simulink model "swingup_polplacement"  (R2020b)
settings: Solver=ode1  StartTime=0.0  StopTime=40  FixedStep=0.01  RelTol=1e-3  EnableMultiTasking=on
values from neighbouring files (symbols this model uses):
  A = A-B*K    [DCMotorODE_up.m]    (also in upright_polplacement.m = [0 0 1 0)
  B = -km * Bold / Rm*gain    [DCMotorODE_up.m]    (also in upright_polplacement.m)
  C = eye(2,4)    [DCMotorODE_up.m]    (also in upright_polplacement.m)
  D = [0;0]    [DCMotorODE_up.m]    (also in upright_polplacement.m = zeros(2,1))
  g = 9.81    [DCMotorODE_up.m]    (also in upright_polplacement.m)
  h = 0.01    [DCMotorODE_up.m]    (also in upright_polplacement.m)
  Jp = mp*Lp^2/3    (= 0.000133128)    [DCMotorODE_up.m]    (also in upright_polplacement.m)
  ke = 0.1    [upright_polplacement.m]
  kt = 0.042    [DCMotorODE_up.m]    (also in upright_polplacement.m)
  l = Lp/2    (= 0.0645)    [DCMotorODE_up.m]    (also in upright_polplacement.m)
  mp = 0.024    [DCMotorODE_up.m]    (also in upright_polplacement.m)
  mr = 0.095    [DCMotorODE_up.m]    (also in upright_polplacement.m)
  r = 0.085    [DCMotorODE_up.m]    (also in upright_polplacement.m)
  Rm = 8.4    [DCMotorODE_up.m]    (also in upright_polplacement.m)
  u_max = 10    [upright_polplacement.m]
undefined symbols (not defined in the file or in its folder): Continuous, Humusoft, K, MF634, Time
libraries: simulink_extras x4, simulink x4, sldrtlib x2, ctrlSharedLib x1, eeLuenbergerObserver x1
settings Model: Creator=rbabuska  LastModifiedBy=zhehanli
settings DataIOCC: LimitDataPoints=on  SaveFormat=Array  SignalLoggingSaveFormat=ModelDataLogs  ReturnWorkspaceOutputs=off
settings OptimizationCC: ExpressionDepthLimit=2147483647  LifeSpan=inf
settings DebuggingCC: UnderspecifiedInitializationDetection=Classic  MergeDetectMultiDrivingBlocksExec=none  FcnCallInpInsideContextMsg=warning  StateNameClashWarn=warning  SFUnexpectedBacktrackingDiag=warning  SFNoUnconditionalDefaultTransitionDiag=warning  SFExecutionAtInitializationDiag=none  ArithmeticOperatorsInVariantConditions=warning
settings HardwareCC: ProdBitPerPointer=32  ProdBitPerSizeT=32  ProdBitPerPtrDiffT=32  ProdLargestAtomicFloat=None  ProdIntDivRoundTo=Undefined  ProdEndianess=Unspecified  ProdWordSize=32  ProdHWDeviceType=32-bit Generic
settings ModelReferenceCC: PropagateSignalLabelsOutOfModel=off
settings SFSimCC: SimUseLocalCustomCode=off  CustomCodeUndefinedFunction=UseInterfaceOnly
settings RTWCC: RTWUseLocalCustomCode=off
settings CodeAppCC: StateflowObjectComments=on
settings GRTTargetCC: TargetLangStandard=C89/C90 (ANSI)  CombineOutputUpdateFcns=off  GRTInterface=on
settings ConfigComp: CovMetricSettings=dw  CovSaveCumulativeToWorkspaceVar=on  CovSaveSingleToWorkspaceVar=on  CovExternalEMLEnable=off  CovSFcnEnable=off

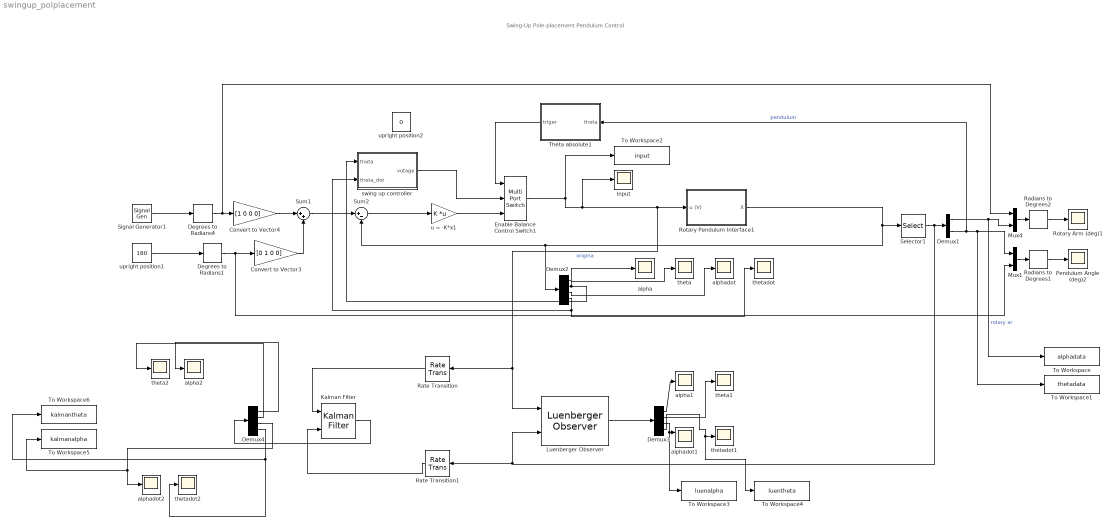
== system swingup_polplacement ==
  note: Swing-Up Pole-placement Pendulum Control
  Convert to Vector3 : Gain  Gain=[0 1 0 0]
  Convert to Vector4 : Gain  Gain=[1 0 0 0]
  Degrees to Radians1 : simulink_extras/Transformations/Degrees to Radians
  Degrees to Radians4 : simulink_extras/Transformations/Degrees to Radians
  Demux1 : Demux  Outputs=2
  Demux2 : Demux
  Demux3 : Demux
  Demux4 : Demux
  Enable Balance Control Switch1 : MultiPortSwitch  DataPortOrder=Zero-based contiguous  Inputs=2  zeroidx=on
  "Input " : Scope
  Kalman Filter : ctrlSharedLib/Kalman Filter  TimeDomain=Continuous-Time  UseCurrentEstimator=on  ModelSource=Individual A, B, C, D matrices  ModelSourceVariable=sys  A=A  B=B  C=C  D=D  NumberOfStates=2  NumberOfInputs=2  NumberOfOutputs=2  InitialEstimateSource=Dialog  X0=[0 0 0 0]  P0=10  UseK=off  UseGH=off  NumberOfProcessNoiseInputs=2  G=1  TimeInvariantG=on  H=0  TimeInvariantH=on  Q=diag([0 0 0.00001 0.00001])  TimeInvariantQ=on  R=0.001  TimeInvariantR=on  N=0  TimeInvariantN=on  AddInputPort=on  AddEnablePort=off  OutputEstimatedY=off  OutputP=off  Ts=h
  Luenberger Observer : eeLuenbergerObserver/Luenberger Observer  StateSpaceType=Continuous-time  Ad=1  Bd=1  Cd=1  Dd=1  A=A  B=B  C=C  D=D  ObserverDesign=Desired eigenvalues  Ld=1  DesiredEigenvalues=[-0.6, -1.5,-10, -20]  x0=[0 0 0 0]  Tsd=0.1  Ts=h
      settings: SourceProductBaseCode=PS
  Mux1 : Mux  Inputs=2
  Mux4 : Mux  Inputs=2
  Pendulum Angle (deg)2 : Scope
  Radians to Degrees1 : simulink_extras/Transformations/Radians to Degrees
  Radians to Degrees2 : simulink_extras/Transformations/Radians to Degrees
  Rate Transition : RateTransition
  Rate Transition1 : RateTransition
  Rotary Arm (deg)1 : Scope
  Rotary Pendulum Interface1 : Subsystem
  Selector1 : Selector  InputPortWidth=4  IndexOptions=Index vector (dialog)  Indices=[1 2]  OutputSizes=1
  Signal Generator1 : SignalGenerator  WaveForm=square  Amplitude=20  Frequency=0.5  Units=rad/sec
  Sum1 : Sum  Inputs=|++
  Sum2 : Sum  Inputs=|+-
  Theta absolute1 : Subsystem
  To Workspace : ToWorkspace  VariableName=alphadata  SaveFormat=Timeseries  SampleTime=h
      settings: Decimation=2
  To Workspace1 : ToWorkspace  VariableName=thetadata  SaveFormat=Timeseries  SampleTime=h
      settings: Decimation=2
  To Workspace2 : ToWorkspace  VariableName=input  SaveFormat=Timeseries  SampleTime=h
      settings: Decimation=2
  To Workspace3 : ToWorkspace  VariableName=luenalpha  SaveFormat=Timeseries  SampleTime=h
      settings: Decimation=2
  To Workspace4 : ToWorkspace  VariableName=luentheta  SaveFormat=Timeseries  SampleTime=h
      settings: Decimation=2
  To Workspace5 : ToWorkspace  VariableName=kalmanalpha  SaveFormat=Timeseries  SampleTime=h
      settings: Decimation=2
  To Workspace6 : ToWorkspace  VariableName=kalmantheta  SaveFormat=Timeseries  SampleTime=h
      settings: Decimation=2
  alpha : Scope
  alpha1 : Scope
  alpha2 : Scope
  alphadot : Scope
  alphadot1 : Scope  NumInputPorts=2
  alphadot2 : Scope
  swing up controller : Subsystem
  theta : Scope
  theta1 : Scope
  theta2 : Scope
  thetadot : Scope
  thetadot1 : Scope
  thetadot2 : Scope
  u = -K*x1 : Gain  Gain=K  Multiplication=Matrix(K*u)
  upright position1 : Constant  Value=180  SampleTime=0
  upright position2 : Constant  Value=0  SampleTime=0
  wires:
  Convert to Vector4/1 -> Sum1/1
  upright position1/1 -> Degrees to Radians1/1
  Demux2/3 -> alphadot/1
  Convert to Vector3/1 -> Sum1/2
  Sum1/1 -> Sum2/1
  u = -K*x1/1 -> Enable Balance Control Switch1/3
  Demux2/1 -> alpha/1
  Degrees to Radians4/1 -> Mux4/1, Convert to Vector4/1
  Radians to Degrees2/1 -> Rotary Arm (deg)1/1
  Demux2/4 -> thetadot/1, swing up controller/2(theta_dot)
  Demux2/2 -> swing up controller/1(theta), theta/1
  Mux1/1 -> Radians to Degrees1/1
  Selector1/1 -> Luenberger Observer/2, Rate Transition1/1, Demux1/1
  Enable Balance Control Switch1/1 -> "Input "/1, Luenberger Observer/1, Rate Transition/1, Rotary Pendulum Interface1/1(u (V)), To Workspace2/1  "origina"
  Rotary Pendulum Interface1/1(X) -> Selector1/1, Demux2/1, Sum2/2
  Signal Generator1/1 -> Degrees to Radians4/1
  Demux1/2 -> To Workspace1/1, Mux1/1, Theta absolute1/1(theta)  "pendulum"
  Radians to Degrees1/1 -> Pendulum Angle (deg)2/1
  Theta absolute1/1(triger) -> Enable Balance Control Switch1/1
  Degrees to Radians1/1 -> Mux1/2, Convert to Vector3/1
  Mux4/1 -> Radians to Degrees2/1
  Demux1/1 -> To Workspace/1, Mux4/2  "rotary ar"
  Sum2/1 -> u = -K*x1/1
  Demux3/4 -> To Workspace4/1, thetadot1/1
  Demux3/2 -> theta1/1
  Demux3/1 -> alpha1/1
  Luenberger Observer/1 -> Demux3/1
  Demux4/3 -> To Workspace5/1, alphadot2/1
  Demux4/4 -> thetadot2/1, To Workspace6/1
  Demux4/2 -> theta2/1
  Demux4/1 -> alpha2/1
  Demux3/3 -> To Workspace3/1, alphadot1/1
  Rate Transition/1 -> Kalman Filter/1
  Rate Transition1/1 -> Kalman Filter/2
  Kalman Filter/1 -> Demux4/1
  swing up controller/1(votage) -> Enable Balance Control Switch1/2

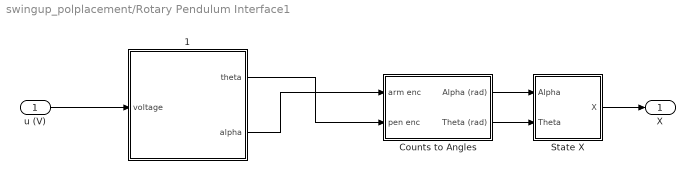
== system swingup_polplacement/Rotary Pendulum Interface1 ==
  u (V) : Inport
  " 1" : Subsystem  LoadFcn=hwinit  InitFcn=hwinit  mask{h=h}
      mask prompts: h "Sampling period [s]"
      mask Display:
      | disp('Qube-Servo')
      | port_label('output',1,'theta')
      | port_label('output',2,'alpha')
      | port_label('input',1,'V')
  Counts to Angles : Subsystem
  State X : Subsystem
  X : Outport  VectorParamsAs1DForOutWhenUnconnected=off
  wires:
  u (V)/1 -> " 1"/1(voltage)
  " 1"/1(theta) -> Counts to Angles/2(pen enc)
  " 1"/2(alpha) -> Counts to Angles/1(arm enc)
  Counts to Angles/2(Theta (rad)) -> State X/2(Theta)
  Counts to Angles/1(Alpha (rad)) -> State X/1(Alpha)
  State X/1(X) -> X/1

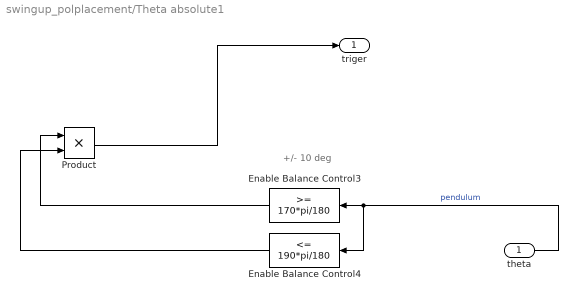
== system swingup_polplacement/Theta absolute1 ==
  note: +/- 10 deg
  theta : Inport
  Enable Balance Control3 : simulink/Logic and Bit Operations/Compare To Constant  relop=>=  const=170*pi/180  OutDataTypeStr=uint8  ZeroCross=off
  Enable Balance Control4 : simulink/Logic and Bit Operations/Compare To Constant  relop=<=  const=190*pi/180  OutDataTypeStr=uint8  ZeroCross=off
  Product : Product
  triger : Outport  VectorParamsAs1DForOutWhenUnconnected=off
  wires:
  Enable Balance Control3/1 -> Product/1
  theta/1 -> Enable Balance Control4/1, Enable Balance Control3/1  "pendulum"
  Enable Balance Control4/1 -> Product/2
  Product/1 -> triger/1

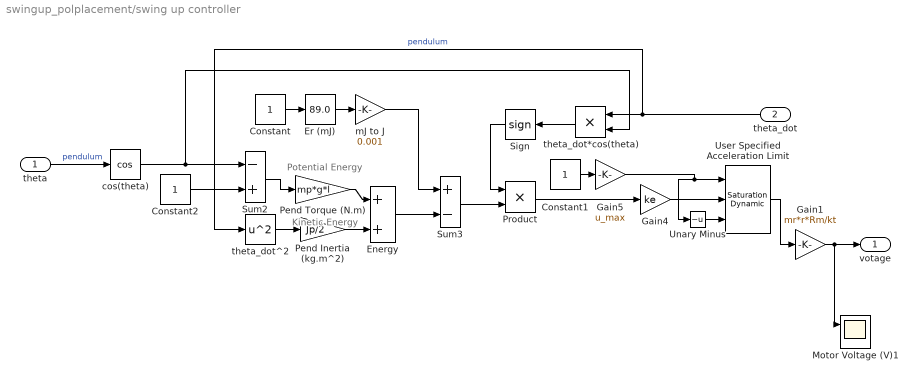
== system swingup_polplacement/swing up controller ==
  note: Kinetic Energy
  note: Potential Energy
  theta : Inport
  theta_dot : Inport  Port=2
  Constant : Constant
  Constant1 : Constant
  Constant2 : Constant
  Energy : Sum  SaturateOnIntegerOverflow=on
  Er (mJ) : simulink/Math Operations/Slider Gain  gain=89.0  low=0  high=100
  Gain1 : Gain  Gain=mr*r*Rm/kt
  Gain4 : Gain  Gain=ke
  Gain5 : Gain  Gain=u_max
  Motor Voltage (V)1 : Scope  NumInputPorts=2
  Pend Inertia (kg.m^2) : Gain  Gain=Jp/2
  Pend Torque (N.m) : Gain  Gain=mp*g*l
  Product : Product  RndMeth=Zero
  Sign : Signum
  Sum2 : Sum  Inputs=-+  SaturateOnIntegerOverflow=on
  Sum3 : Sum  Inputs=+-  SaturateOnIntegerOverflow=on
  Unary Minus : UnaryMinus
  User Specified Acceleration Limit : simulink/Discontinuities/Saturation Dynamic  OutMin=-u_max  OutMax=u_max  OutDataTypeStr=Inherit: Same as second input  OutDataType=fixdt(1, 16)  OutScaling=2^-10  DoSatur=off
  cos(theta) : Trigonometry  Operator=cos
  mJ to J : Gain  Gain=0.001
  theta_dot*cos(theta) : Product  RndMeth=Zero
  theta_dot^2 : Math  Operator=square  SignedPower=on  SaturateOnIntegerOverflow=on
  votage : Outport  VectorParamsAs1DForOutWhenUnconnected=off
  wires:
  Gain5/1 -> Unary Minus/1, User Specified Acceleration Limit/1
  Constant1/1 -> Gain5/1
  Er (mJ)/1 -> mJ to J/1
  User Specified Acceleration Limit/1 -> Gain1/1
  Energy/1 -> Sum3/2
  theta_dot*cos(theta)/1 -> Sign/1
  Constant2/1 -> Sum2/2
  Sum2/1 -> Pend Torque (N.m)/1
  Pend Torque (N.m)/1 -> Energy/1
  theta_dot^2/1 -> Pend Inertia (kg.m^2)/1
  Sum3/1 -> Product/2
  Product/1 -> Gain4/1
  Gain1/1 -> Motor Voltage (V)1/1, votage/1
  Sign/1 -> Product/1
  Constant/1 -> Er (mJ)/1
  Unary Minus/1 -> User Specified Acceleration Limit/3
  Gain4/1 -> User Specified Acceleration Limit/2
  Pend Inertia (kg.m^2)/1 -> Energy/2
  mJ to J/1 -> Sum3/1
  theta/1 -> cos(theta)/1  "pendulum"
  cos(theta)/1 -> theta_dot*cos(theta)/2, Sum2/1
  theta_dot/1 -> theta_dot^2/1, theta_dot*cos(theta)/1  "pendulum"

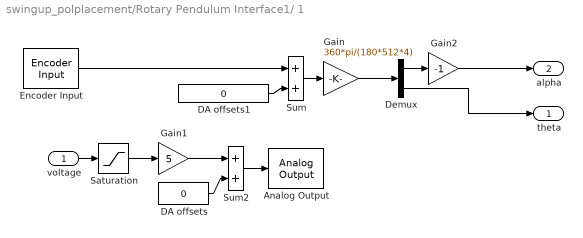
== system swingup_polplacement/Rotary Pendulum Interface1/ 1 ==
  voltage : Inport
  Analog Output : sldrtlib/Analog Output  SampleTime=h  MaxMissedTicks=100  ShowMissedTicks=off  YieldWhenWaiting=off  DrvName=Humusoft/MF634  DrvAddress=4294967295  DrvOptions=0  Channels=[1]  RangeMode=2  VoltRange=1  InitialValue=0  FinalValue=0
      settings: AttributesFormatString=Humusoft\nMF634 [auto]
  DA offsets : Constant  Value=0
  DA offsets1 : Constant  Value=0  SampleTime=h
  Demux : Demux  Outputs=2
  Encoder Input : sldrtlib/Encoder Input  SampleTime=h  MaxMissedTicks=100  ShowMissedTicks=off  YieldWhenWaiting=off  DrvName=Humusoft/MF634  DrvAddress=4294967295  DrvOptions=0  Channels=[1,2]  QuadMode=3  IndexPulse=1  InputFilter=Inf  DataType=1
      settings: AttributesFormatString=Humusoft\nMF634 [auto]
  Gain : Gain  Gain=360*pi/(180*512*4)  SaturateOnIntegerOverflow=on  OutDataTypeStr=Inherit: Same as input  ParamDataTypeStr=Inherit: Same as input
  Gain1 : Gain  Gain=5  SaturateOnIntegerOverflow=on  OutDataTypeStr=Inherit: Same as input  ParamDataTypeStr=Inherit: Same as input
  Gain2 : Gain  Gain=-1  SaturateOnIntegerOverflow=on  OutDataTypeStr=Inherit: Same as input  ParamDataTypeStr=Inherit: Same as input
  Saturation : Saturate  UpperLimit=1  LowerLimit=-1
  Sum : Sum  InputSameDT=on  SaturateOnIntegerOverflow=on  OutDataTypeStr=Inherit: Same as first input
  Sum2 : Sum  InputSameDT=on  SaturateOnIntegerOverflow=on  OutDataTypeStr=Inherit: Same as first input
  theta : Outport  Tag=Cable length
  alpha : Outport  Tag=Cable length  Port=2
  wires:
  Sum/1 -> Gain/1
  DA offsets1/1 -> Sum/2
  Gain1/1 -> Sum2/1
  Sum2/1 -> Analog Output/1
  DA offsets/1 -> Sum2/2
  voltage/1 -> Saturation/1
  Encoder Input/1 -> Sum/1
  Saturation/1 -> Gain1/1
  Demux/1 -> Gain2/1
  Gain/1 -> Demux/1
  Gain2/1 -> alpha/1
  Demux/2 -> theta/1

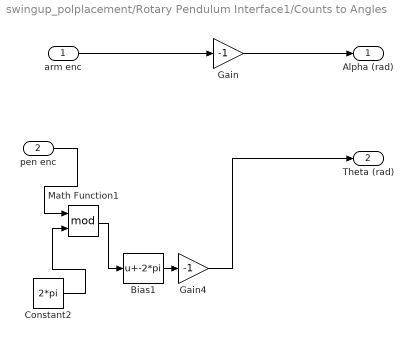
== system swingup_polplacement/Rotary Pendulum Interface1/Counts to Angles ==
  arm enc : Inport
  pen enc : Inport  Port=2
  Bias1 : Bias  Bias=-2*pi
  Constant2 : Constant  Value=2*pi
  Gain : Gain  Gain=-1
  Gain4 : Gain  Gain=-1
  Math Function1 : Math  Operator=mod  SignedPower=on  SaturateOnIntegerOverflow=on
  Alpha (rad) : Outport  VectorParamsAs1DForOutWhenUnconnected=off
  Theta (rad) : Outport  Port=2  VectorParamsAs1DForOutWhenUnconnected=off
  wires:
  arm enc/1 -> Gain/1
  Gain4/1 -> Theta (rad)/1
  Math Function1/1 -> Bias1/1
  pen enc/1 -> Math Function1/1
  Constant2/1 -> Math Function1/2
  Bias1/1 -> Gain4/1
  Gain/1 -> Alpha (rad)/1

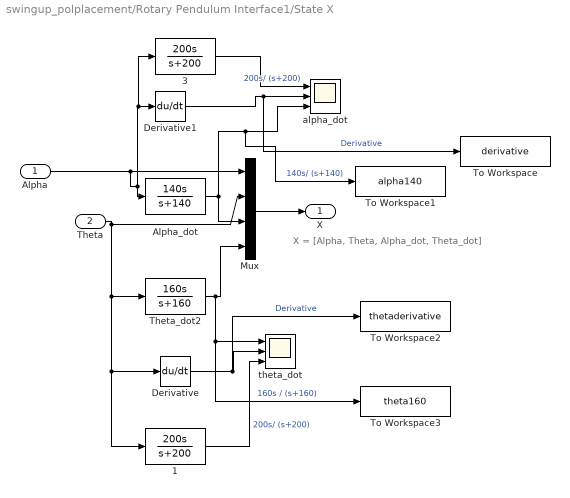
== system swingup_polplacement/Rotary Pendulum Interface1/State X ==
  note: X = [Alpha, Theta, Alpha_dot, Theta_dot]
  Alpha : Inport
  Theta : Inport  Port=2
  1 : TransferFcn  Numerator=[200 0]  Denominator=[1 200]
  3 : TransferFcn  Numerator=[200 0]  Denominator=[1 200]
  Alpha_dot : TransferFcn  Numerator=[140 0]  Denominator=[1 140]
  Derivative : Derivative
  Derivative1 : Derivative
  Mux : Mux
  Theta_dot2 : TransferFcn  Numerator=[160 0]  Denominator=[1 160]
  To Workspace : ToWorkspace  VariableName=derivative  SaveFormat=Timeseries  SampleTime=h
      settings: Decimation=2
  To Workspace1 : ToWorkspace  VariableName=alpha140  SaveFormat=Timeseries  SampleTime=h
      settings: Decimation=2
  To Workspace2 : ToWorkspace  VariableName=thetaderivative  SaveFormat=Timeseries  SampleTime=h
      settings: Decimation=2
  To Workspace3 : ToWorkspace  VariableName=theta160  SaveFormat=Timeseries  SampleTime=h
      settings: Decimation=2
  alpha_dot : Scope  NumInputPorts=3
  theta_dot : Scope  NumInputPorts=3
  X : Outport  VectorParamsAs1DForOutWhenUnconnected=off
  wires:
  Alpha_dot/1 -> Mux/3, To Workspace1/1, alpha_dot/3  "140s/ (s+140)"
  Mux/1 -> X/1
  Alpha/1 -> Mux/1, 3/1, Derivative1/1, Alpha_dot/1
  Theta_dot2/1 -> To Workspace3/1, theta_dot/1, Mux/4  "160s / (s+160)"
  Derivative/1 -> To Workspace2/1, theta_dot/2  "Derivative"
  Theta/1 -> Mux/2, Theta_dot2/1, Derivative/1, 1/1
  1/1 -> theta_dot/3  "200s/ (s+200)"
  3/1 -> alpha_dot/1  "200s/ (s+200)"
  Derivative1/1 -> To Workspace/1, alpha_dot/2  "Derivative"
